simulink model "DataAcquisition_RPM"  (R2022b)
settings: Solver=FixedStepAuto  StartTime=0.0  StopTime=20  FixedStep=Ts  RelTol=1e-3
model workspace (MAT data in the model file):
  Ts = 0.1
libraries: arduinolib x4, SignalEditorBlockLib x2
settings Model: SimulationMode=external  ExtModeTrigDuration=2  Creator=Prashanth  LastModifiedBy=Prashanth
settings OptimizationCC: EnhancedBackFolding=on  PassReuseOutputArgsAs=Individual arguments  ZeroExternalMemoryAtStartup=off  ZeroInternalMemoryAtStartup=off  MaxStackSize=64  OptimizeBlockOrder=speed  DifferentSizesBufferReuse=on  OptimizationCustomize=off  EfficientTunableParamExpr=on
settings DebuggingCC: ParameterTunabilityLossMsg=error
settings HardwareCC: ProdBitPerInt=16  ProdBitPerPointer=16  ProdBitPerSizeT=16  ProdBitPerPtrDiffT=16  ProdLargestAtomicFloat=None  ProdWordSize=8  ProdHWDeviceType=Atmel->AVR
settings SFSimCC: MATLABDynamicMemAlloc=off
settings RTWCC: Description=Embedded Coder  SystemTargetFile=ert.tlc  HardwareBoard=Arduino Mega 2560  TLCOptions=-aInlineSetEventsForThisBaseRateFcn=TLC_FALSE -aSuppressMultiTaskScheduler=TLC_FALSE -aRateBasedStepFcn=1  TemplateMakefile=ert_default_tmf  Toolchain=Arduino AVR
settings CodeAppCC: ForceParamTrailComments=on  IgnoreCustomStorageClasses=off  OperatorAnnotations=on  SimulinkDataObjDesc=on  SFDataObjDesc=on  InsertBlockDesc=on
settings ERTTargetCC: SupportContinuousTime=on  SupportVariableSizeSignals=on  ExtModeTransport=3  ExtModeStaticAlloc=on  ExtModeAutomaticAllocSize=off  ExtModeStaticAllocSize=2048  ExtModeMexFile=ext_xcp  ExtModeIntrfLevel=Level2 - Open

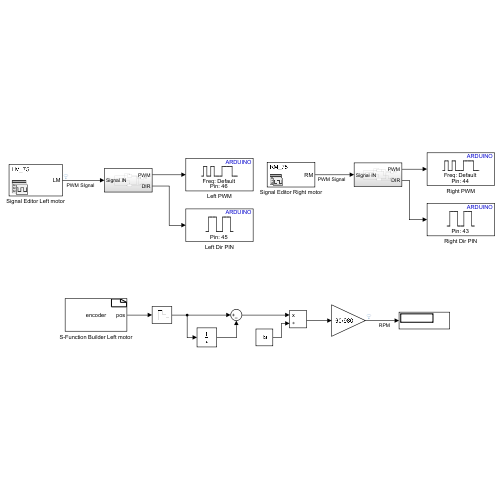
[thumbnail: Simulink's stored preview of the top-level diagram]
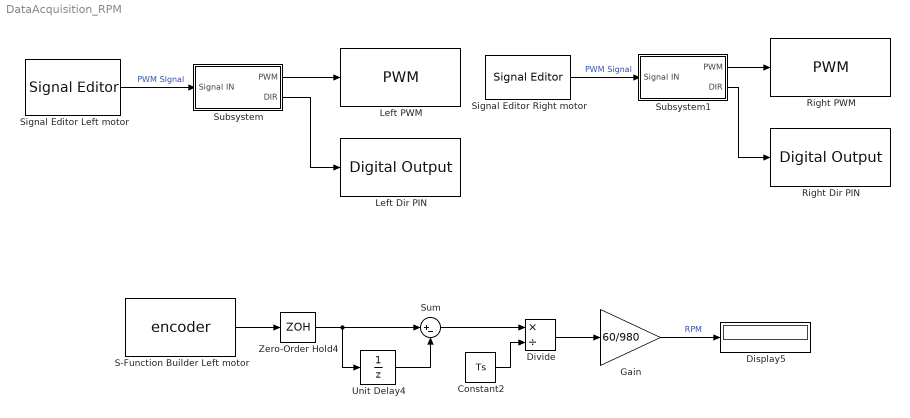
== system DataAcquisition_RPM ==
  Constant2 : Constant  Value=Ts  SampleTime=Ts
  Display5 : Display
  Divide : Product  Inputs=*/
  Gain : Gain  Gain=60/980
  Left Dir PIN : arduinolib/Digital Output  pinNumber=45  Direction=output  blockPlatform=arduino
  Left PWM : arduinolib/PWM  pinNumber=46  frequencyType=Default  desiredFrequency=490.2  achievableFrequency=490.2
  Right Dir PIN : arduinolib/Digital Output  pinNumber=43  Direction=output  blockPlatform=arduino
  Right PWM : arduinolib/PWM  pinNumber=44  frequencyType=Default  desiredFrequency=640000  achievableFrequency=615384.6154
  S-Function Builder Left motor : S-Function  InitFcn=try, set_param(gcb,'FunctionName','encoder'), end  FunctionName=encoder  Parameters=int8(0),int8(18),int8(19)  SFunctionModules=encoder_wrapper.c  SFunctionDeploymentMode=off  EnableBusSupport=off  mask(S-Function Builder){}
      mask help: Simulink:masks:SFunctionBuilder_MD
      mask init:
      | val = [[.9  0.75 0.75 1 1 .9 .9 1]',[1 1 0.75 0.75 .9 .9 1 .9]'];try , sys = get_param(gcb,'SfunBuilderFcnName');if isempty(sys), sys = get_param(gcb,'FunctionName'); end,catch, sys = get_param(gcb,'FunctionName'); end
      settings: CopyFcn=set_param(gcbh,'LinkStatus','none')  PreSaveFcn=try, set_param(gcb,'FunctionName','encoder'), end  OpenFcn=sfunctionwizard(gcbh)
      mask Display: plot(val(:,1),val(:,2)),disp(sys), port_label('output',1,'pos')
  Signal Editor Left motor : SignalEditorBlockLib/Signal Editor  FileName=PWM_Signals.mat  ActiveScenario=LM_75  ActiveSignal=LM  IsBus=off  OutputBusObjectStr=Bus: BusObject  SampleTime=0  Interpolate=off  ZeroCross=off  OutputAfterFinalValue=Setting to zero  Unit=inherit  PreserveSignalName=on
  Signal Editor Right motor : SignalEditorBlockLib/Signal Editor  FileName=PWM_Signals.mat  ActiveScenario=RM_75  ActiveSignal=RM  IsBus=off  OutputBusObjectStr=Bus: BusObject  SampleTime=0  Interpolate=off  ZeroCross=off  OutputAfterFinalValue=Setting to zero  Unit=inherit  PreserveSignalName=on
  Subsystem : Subsystem
  Subsystem1 : Subsystem
  Sum : Sum  Inputs=|+-
  Unit Delay4 : UnitDelay  SampleTime=-1  HasFrameUpgradeWarning=on
  Zero-Order Hold4 : ZeroOrderHold  SampleTime=Ts
  wires:
  Signal Editor Left motor/1 -> Subsystem/1(Signal IN)  "PWM SIgnal"
  Gain/1 -> Display5/1  "RPM"
  Constant2/1 -> Divide/2
  Unit Delay4/1 -> Sum/2
  Divide/1 -> Gain/1
  Sum/1 -> Divide/1
  S-Function Builder Left motor/1 -> Zero-Order Hold4/1
  Zero-Order Hold4/1 -> Sum/1, Unit Delay4/1
  Subsystem/1(PWM) -> Left PWM/1
  Subsystem/2(DIR) -> Left Dir PIN/1
  Subsystem1/2(DIR) -> Right Dir PIN/1
  Subsystem1/1(PWM) -> Right PWM/1
  Signal Editor Right motor/1 -> Subsystem1/1(Signal IN)  "PWM Signal"

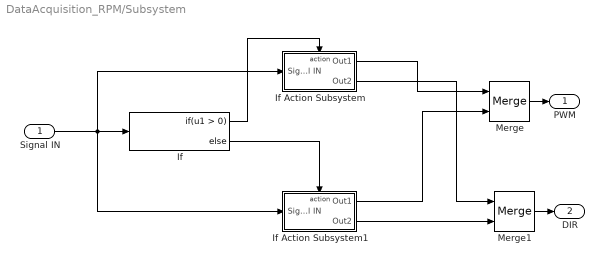
== system DataAcquisition_RPM/Subsystem ==
  Signal IN : Inport
  If : If
  If Action Subsystem : Subsystem  TreatAsAtomicUnit=on
  If Action Subsystem1 : Subsystem  TreatAsAtomicUnit=on
  Merge : Merge
  Merge1 : Merge
  PWM : Outport
  DIR : Outport  Port=2
  wires:
  Signal IN/1 -> If Action Subsystem/1(Signal IN), If Action Subsystem1/1(Signal IN), If/1
  If/2 -> If Action Subsystem1/Action
  If/1 -> If Action Subsystem/Action
  If Action Subsystem/1(Out1) -> Merge/1
  If Action Subsystem1/1(Out1) -> Merge/2
  If Action Subsystem1/2(Out2) -> Merge1/2
  If Action Subsystem/2(Out2) -> Merge1/1
  Merge1/1 -> DIR/1
  Merge/1 -> PWM/1

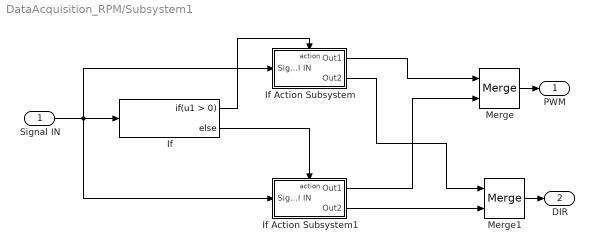
== system DataAcquisition_RPM/Subsystem1 ==
  Signal IN : Inport
  If : If
  If Action Subsystem : Subsystem  TreatAsAtomicUnit=on
  If Action Subsystem1 : Subsystem  TreatAsAtomicUnit=on
  Merge : Merge
  Merge1 : Merge
  PWM : Outport
  DIR : Outport  Port=2
  wires:
  Merge/1 -> PWM/1
  Merge1/1 -> DIR/1
  If Action Subsystem/2(Out2) -> Merge1/1
  If Action Subsystem1/2(Out2) -> Merge1/2
  If Action Subsystem1/1(Out1) -> Merge/2
  If Action Subsystem/1(Out1) -> Merge/1
  If/1 -> If Action Subsystem/Action
  If/2 -> If Action Subsystem1/Action
  Signal IN/1 -> If Action Subsystem/1(Signal IN), If Action Subsystem1/1(Signal IN), If/1

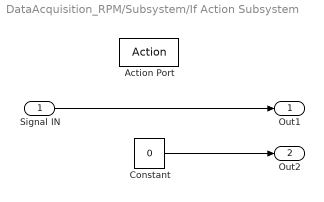
== system DataAcquisition_RPM/Subsystem/If Action Subsystem ==
  Signal IN : Inport
  Action Port : ActionPort  ActionPortLabel=if(u1 > 0)
  Constant : Constant  Value=0
  Out1 : Outport
  Out2 : Outport  Port=2
  wires:
  Signal IN/1 -> Out1/1
  Constant/1 -> Out2/1

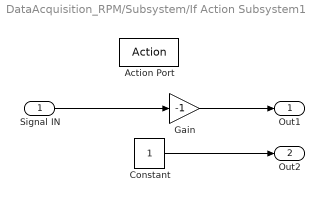
== system DataAcquisition_RPM/Subsystem/If Action Subsystem1 ==
  Signal IN : Inport
  Action Port : ActionPort  ActionPortLabel=else
  Constant : Constant
  Gain : Gain  Gain=-1
  Out1 : Outport
  Out2 : Outport  Port=2
  wires:
  Signal IN/1 -> Gain/1
  Constant/1 -> Out2/1
  Gain/1 -> Out1/1

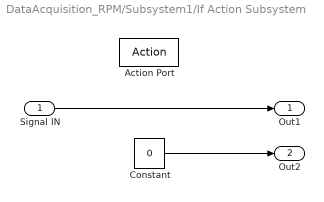
== system DataAcquisition_RPM/Subsystem1/If Action Subsystem ==
  Signal IN : Inport
  Action Port : ActionPort  ActionPortLabel=if(u1 > 0)
  Constant : Constant  Value=0
  Out1 : Outport
  Out2 : Outport  Port=2
  wires:
  Constant/1 -> Out2/1
  Signal IN/1 -> Out1/1

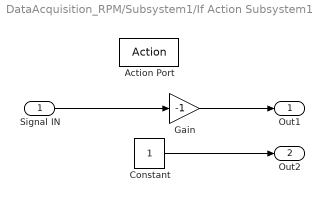
== system DataAcquisition_RPM/Subsystem1/If Action Subsystem1 ==
  Signal IN : Inport
  Action Port : ActionPort  ActionPortLabel=else
  Constant : Constant
  Gain : Gain  Gain=-1
  Out1 : Outport
  Out2 : Outport  Port=2
  wires:
  Gain/1 -> Out1/1
  Constant/1 -> Out2/1
  Signal IN/1 -> Gain/1
